simulink model "Traffic_Light_ROS2_demo"  (R2024b)
settings: Solver=FixedStepAuto  StartTime=0.0  StopTime=60  FixedStep=0.1  MaxStep=0.05  RelTol=1e-3
model workspace (MAT data in the model file):
  SL_ROS_VariableLengthArrays_MaxSizes : object (value not decoded)
undefined symbols (not defined in the file or in its folder): brake, gear, hand_brake, manual_gear_shift, reverse, steer, throttle
libraries: ros2lib x9, visionsinks x1
(part 2 of 2)

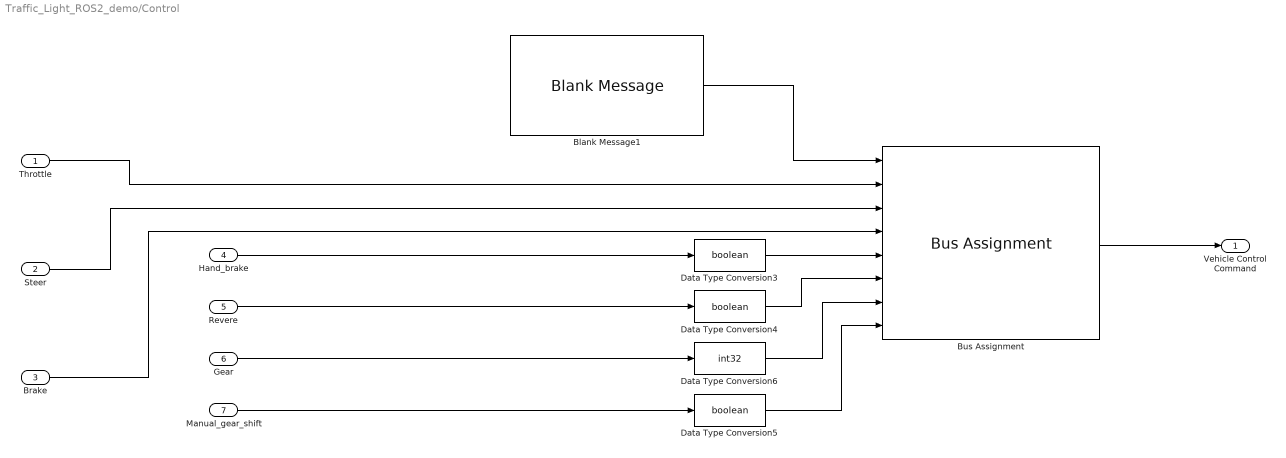
== system Traffic_Light_ROS2_demo/Control ==
  Throttle : Inport
  Steer : Inport  Port=2
  Brake : Inport  Port=3
  Hand_brake : Inport  Port=4
  Revere : Inport  Port=5
  Gear : Inport  Port=6
  Manual_gear_shift : Inport  Port=7
  Blank Message1 : ros2lib/Blank Message  messageClass=Message  entityType=carla_msgs/CarlaEgoVehicleControl  messageType=carla_msgs/CarlaEgoVehicleControl  SampleTime=inf
  Bus Assignment : BusAssignment  AssignedSignals=throttle,steer,brake,hand_brake,reverse,gear,manual_gear_shift
  Data Type Conversion3 : DataTypeConversion  OutDataTypeStr=boolean  SaturateOnIntegerOverflow=off  RndMeth=Floor
  Data Type Conversion4 : DataTypeConversion  OutDataTypeStr=boolean  SaturateOnIntegerOverflow=off  RndMeth=Floor
  Data Type Conversion5 : DataTypeConversion  OutDataTypeStr=boolean  SaturateOnIntegerOverflow=off  RndMeth=Floor
  Data Type Conversion6 : DataTypeConversion  OutDataTypeStr=int32  SaturateOnIntegerOverflow=off  RndMeth=Floor
  Vehicle Control Command : Outport
  wires:
  Data Type Conversion5/1 -> Bus Assignment/8
  Data Type Conversion6/1 -> Bus Assignment/7
  Blank Message1/1 -> Bus Assignment/1
  Data Type Conversion4/1 -> Bus Assignment/6
  Data Type Conversion3/1 -> Bus Assignment/5
  Throttle/1 -> Bus Assignment/2
  Manual_gear_shift/1 -> Data Type Conversion5/1
  Bus Assignment/1 -> Vehicle Control Command/1
  Revere/1 -> Data Type Conversion4/1
  Steer/1 -> Bus Assignment/3
  Brake/1 -> Bus Assignment/4
  Hand_brake/1 -> Data Type Conversion3/1
  Gear/1 -> Data Type Conversion6/1

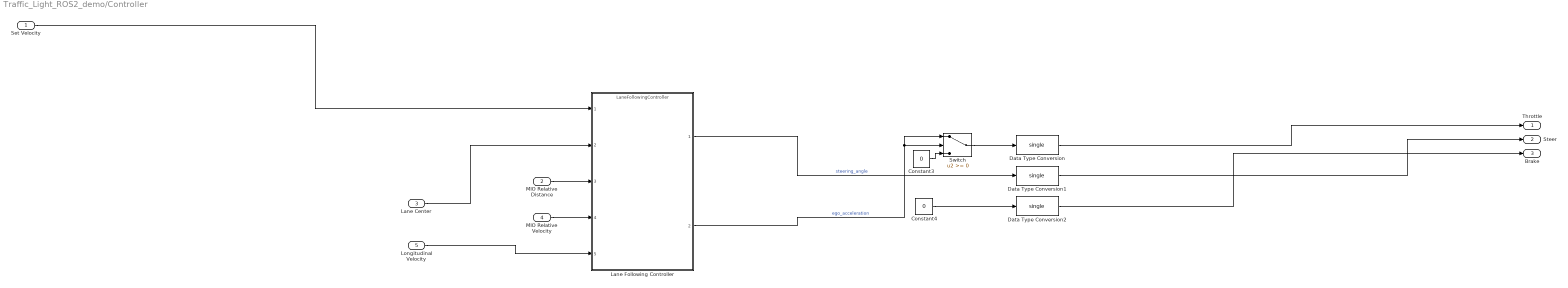
== system Traffic_Light_ROS2_demo/Controller ==
  Set Velocity : Inport
  MIO Relative Distance : Inport  Port=2
  Lane Center : Inport  Port=3
  MIO Relative Velocity : Inport  Port=4
  Longitudinal Velocity : Inport  Port=5
  Constant3 : Constant  Value=0
  Constant4 : Constant  Value=0
  Data Type Conversion : DataTypeConversion  OutDataTypeStr=single  SaturateOnIntegerOverflow=off  RndMeth=Floor
  Data Type Conversion1 : DataTypeConversion  OutDataTypeStr=single  SaturateOnIntegerOverflow=off  RndMeth=Floor
  Data Type Conversion2 : DataTypeConversion  OutDataTypeStr=single  SaturateOnIntegerOverflow=off  RndMeth=Floor
  Lane Following Controller : ModelReference  ModelNameDialog=LaneFollowingController  SimulationMode=Normal  CodeInterface=Top model  ModelReferenceVersion=10.13
  Switch : Switch  SaturateOnIntegerOverflow=off  InputSameDT=off
  Throttle : Outport
  Steer : Outport  Port=2
  Brake : Outport  Port=3
  wires:
  Set Velocity/1 -> Lane Following Controller/1
  Longitudinal Velocity/1 -> Lane Following Controller/5
  Constant3/1 -> Switch/3
  Lane Following Controller/1 -> Data Type Conversion1/1  "steering_angle"
  Data Type Conversion2/1 -> Brake/1
  MIO Relative Velocity/1 -> Lane Following Controller/4
  Data Type Conversion1/1 -> Steer/1
  Lane Center/1 -> Lane Following Controller/2
  Switch/1 -> Data Type Conversion/1
  Constant4/1 -> Data Type Conversion2/1
  MIO Relative Distance/1 -> Lane Following Controller/3
  Lane Following Controller/2 -> Switch/1, Switch/2  "ego_acceleration"
  Data Type Conversion/1 -> Throttle/1

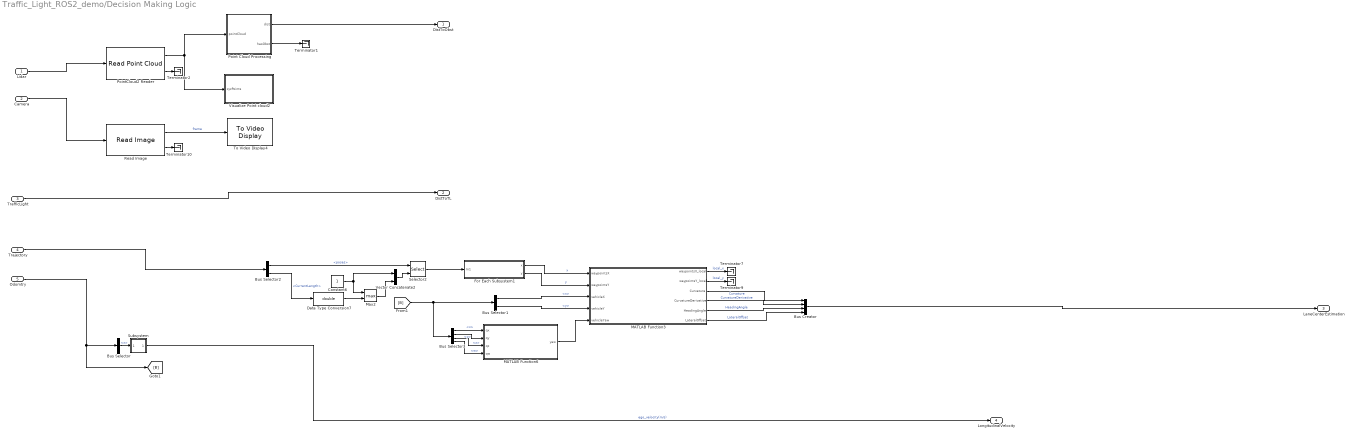
== system Traffic_Light_ROS2_demo/Decision Making Logic ==
  Lidar : Inport
  Camera : Inport  Port=2
  TrafficLight : Inport  Port=3
  Trajectory : Inport  Port=4
  Odomtry : Inport  Port=5
  Bus Creator : BusCreator  Inputs=4
  Bus Selector : BusSelector  OutputSignals=twist.twist.linear.x
  Bus Selector1 : BusSelector  OutputSignals=pose.pose.position.x,pose.pose.position.y
  Bus Selector2 : BusSelector  OutputSignals=poses,poses_SL_Info.CurrentLength
  Bus Selector3 : BusSelector  OutputSignals=pose.pose.orientation.x,pose.pose.orientation.y,pose.pose.orientation.z,pose.pose.orientation.w
  Constant6 : Constant  SampleTime=-1
  Data Type Conversion7 : DataTypeConversion  OutDataTypeStr=double  SaturateOnIntegerOverflow=off  RndMeth=Floor
  For Each Subsystem1 : Subsystem  TreatAsAtomicUnit=on
  MATLAB Function3 : MATLAB Function  TreatAsAtomicUnit=on
  MATLAB Function6 : MATLAB Function  TreatAsAtomicUnit=on
  Max2 : MinMax  Function=max  Inputs=2
  Point Cloud Processing : Subsystem
  PointCloud2 Reader : ros2lib/Read Point Cloud  MaximumPointCloudSize=[1, 8292]  PreserveStructure=off  ShowRGBOutput=off  ShowIntensityOutput=off  ShowErrorCodeOutput=on  VariableSizeOutputs=off
  Read Image : ros2lib/Read Image  MaximumImageSize=[600, 800]  ImageEncoding=bgra8  ShowAlphaOutput=off  ShowErrorCodeOutput=on  VariableSizeOutputs=off
  Selector2 : Selector  IndexOptions=Starting and ending indices (port)  Indices=1  OutputSizes=1  RuntimeRangeChecks=on
  Subsystem : Subsystem
  Terminator{1..2,7,9..10} (5 alike) : Terminator
  To Video Display4 : visionsinks/To Video Display  windowSizeMode=Normal  openAtMdlStart=on  fullScreen=off  videoWindowX=536805376  videoWindowY=536805376  saveWindowSize=off  videoWindowWidth=1395  videoWindowHeight=752  inputColorFormat=RGB  inputType=Obsolete  imagePorts=One multidimensional signal  OutputDevice=On-screen video monitor  dataOrg=Column-major  isWindowOpen=off
  Vector Concatenate2 : Concatenate
  Visualize Point cloud2 : MATLAB Function  StopFcn=|  TreatAsAtomicUnit=on
      | playerFigure = findall(groot,'type','figure','name','Point Cloud Player');
      | 
      | if ~isempty(playerFigure)
      |     playerFigure = playerFigure(end);
      |     if isvalid(playerFigure)
      |         close(playerFigure);
      |     end
      | end
  DistToObst : Outport
  DistToTL : Outport  Port=2
  LaneCenterEstimation : Outport  Port=3
  LongitudinalVelocity : Outport  Port=4
  wires:
  MATLAB Function3/5(HeadingAngle) -> Bus Creator/3  "HeadingAngle"
  Read Image/2 -> Terminator10/1
  Subsystem/1(Out1) -> LongitudinalVelocity/1  "ego_velocity(m/s)"
  PointCloud2 Reader/2 -> Terminator2/1
  MATLAB Function3/3(Curvature) -> Bus Creator/1  "Curvature"
  Bus Selector3/1 -> MATLAB Function6/1(qx)  "<x>"
  PointCloud2 Reader/1 -> Visualize Point cloud2/1(xyzPoints), Point Cloud Processing/1(pointCloud)
  Odomtry/1 -> [B], Bus Selector/1
  Constant6/1 -> Vector Concatenate2/1, Max2/1
  Read Image/1 -> To Video Display4/1  "frame"
  Data Type Conversion7/1 -> Max2/2
  For Each Subsystem1/1(x) -> MATLAB Function3/1(waypointsX)  "x"
  Bus Selector2/1 -> Selector2/1  "<poses>"
  Bus Selector3/3 -> MATLAB Function6/3(qz)  "<z>"
  Bus Selector2/2 -> Data Type Conversion7/1  "<CurrentLength>"
  Point Cloud Processing/2(hasObst) -> Terminator1/1
  MATLAB Function3/6(LateralOffset) -> Bus Creator/4  "LateralOffset"
  Trajectory/1 -> Bus Selector2/1
  Bus Selector3/4 -> MATLAB Function6/4(qw)  "<w>"
  Selector2/1 -> For Each Subsystem1/1(In1)
  MATLAB Function3/2(waypointsY_local) -> Terminator9/1  "local_y"
  Lidar/1 -> PointCloud2 Reader/1
  MATLAB Function6/1(yaw) -> MATLAB Function3/5(vehicleYaw)
  Point Cloud Processing/1(dist) -> DistToObst/1
  Camera/1 -> Read Image/1
  Bus Selector3/2 -> MATLAB Function6/2(qy)  "<y>"
  Vector Concatenate2/1 -> Selector2/2
  [B] -> Bus Selector1/1, Bus Selector3/1
  Bus Selector1/2 -> MATLAB Function3/4(vehicleY)  "<y>"
  Bus Creator/1 -> LaneCenterEstimation/1
  MATLAB Function3/1(waypointsX_local) -> Terminator7/1  "local_x"
  Bus Selector/1 -> Subsystem/1(In1)  "<x>"
  Max2/1 -> Vector Concatenate2/2
  MATLAB Function3/4(CurvatureDerivative) -> Bus Creator/2  "CurvatureDerivative"
  For Each Subsystem1/2(y) -> MATLAB Function3/2(waypointsY)  "y"
  Bus Selector1/1 -> MATLAB Function3/3(vehicleX)  "<x>"
  TrafficLight/1 -> DistToTL/1

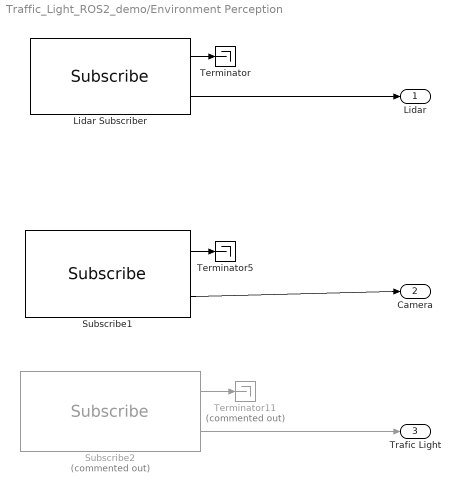
== system Traffic_Light_ROS2_demo/Environment Perception ==
  Lidar Subscriber : ros2lib/Subscribe  topicSource=Select from ROS network  topic=/carla/hero/lidar  messageType=sensor_msgs/PointCloud2  sampleTime=-1  QOSHistory=Keep last  QOSDepth=1  QOSReliability=Reliable  QOSDurability=Volatile  QOSDeadline=Inf  QOSLifespan=Inf  QOSLiveliness=Automatic  QOSLeaseDuration=Inf  QOSAvoidROSNamespaceConventions=off
  Subscribe1 : ros2lib/Subscribe  topicSource=Select from ROS network  topic=/carla/hero/rgb_front/image  messageType=sensor_msgs/Image  sampleTime=-1  QOSHistory=Keep last  QOSDepth=1  QOSReliability=Reliable  QOSDurability=Volatile  QOSDeadline=Inf  QOSLifespan=Inf  QOSLiveliness=Automatic  QOSLeaseDuration=Inf  QOSAvoidROSNamespaceConventions=off
  Subscribe2 : ros2lib/Subscribe  Commented=on  topicSource=Select from ROS network  topic=/carla/hero/traffic_light_in_front  messageType=carla_msgs/TrafficLightInfo  sampleTime=-1  QOSHistory=Keep last  QOSDepth=1  QOSReliability=Reliable  QOSDurability=Transient local  QOSDeadline=Inf  QOSLifespan=Inf  QOSLiveliness=Automatic  QOSLeaseDuration=Inf  QOSAvoidROSNamespaceConventions=off
  Terminator : Terminator
  Terminator11 : Terminator  Commented=on
  Terminator5 : Terminator
  Lidar : Outport
  Camera : Outport  Port=2
  Trafic Light : Outport  Port=3
  wires:
  Subscribe2/1 -> Terminator11/1
  Lidar Subscriber/1 -> Terminator/1
  Subscribe1/1 -> Terminator5/1
  Subscribe2/2 -> Trafic Light/1
  Lidar Subscriber/2 -> Lidar/1
  Subscribe1/2 -> Camera/1

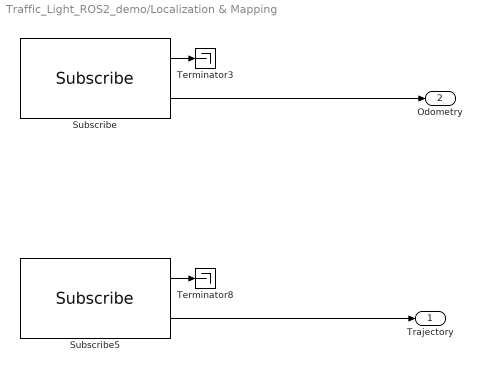
== system Traffic_Light_ROS2_demo/Localization & Mapping ==
  Subscribe : ros2lib/Subscribe  topicSource=Select from ROS network  topic=/carla/hero/odometry  messageType=nav_msgs/Odometry  sampleTime=-1  QOSHistory=Keep last  QOSDepth=1  QOSReliability=Reliable  QOSDurability=Volatile  QOSDeadline=Inf  QOSLifespan=Inf  QOSLiveliness=Automatic  QOSLeaseDuration=Inf  QOSAvoidROSNamespaceConventions=off
  Subscribe5 : ros2lib/Subscribe  topicSource=Select from ROS network  topic=/carla/hero/waypoints  messageType=nav_msgs/Path  sampleTime=-1  QOSHistory=Keep last  QOSDepth=1  QOSReliability=Reliable  QOSDurability=Transient local  QOSDeadline=Inf  QOSLifespan=Inf  QOSLiveliness=Automatic  QOSLeaseDuration=Inf  QOSAvoidROSNamespaceConventions=off
  Terminator3 : Terminator
  Terminator8 : Terminator
  Trajectory : Outport
  Odometry : Outport  Port=2
  wires:
  Subscribe5/1 -> Terminator8/1
  Subscribe/1 -> Terminator3/1
  Subscribe5/2 -> Trajectory/1
  Subscribe/2 -> Odometry/1

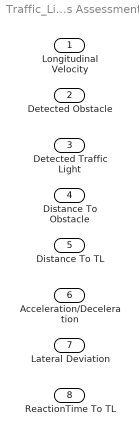
== system Traffic_Light_ROS2_demo/Metrics Assessment ==
  Longitudinal Velocity : Inport
  Detected Obstacle : Inport  Port=2
  Detected Traffic Light : Inport  Port=3
  Distance To Obstacle : Inport  Port=4
  Distance To TL : Inport  Port=5
  Acceleration/Deceleration : Inport  Port=6
  Lateral Deviation : Inport  Port=7
  ReactionTime To TL : Inport  Port=8

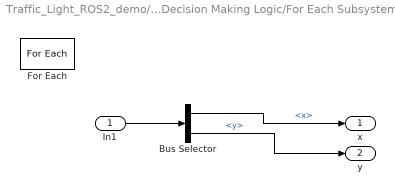
== system Traffic_Light_ROS2_demo/Decision Making Logic/For Each Subsystem1 ==
  In1 : Inport  Partition=on  PartitionDimension=1  PartitionWidth=1  PartitionOffset=0
  Bus Selector : BusSelector  OutputSignals=pose.position.x,pose.position.y
  For Each : ForEach  DisableCoverage=on
  x : Outport  ConcatenationDimension=1
  y : Outport  Port=2  ConcatenationDimension=1
  wires:
  In1/1 -> Bus Selector/1
  Bus Selector/1 -> x/1  "<x>"
  Bus Selector/2 -> y/1  "<y>"

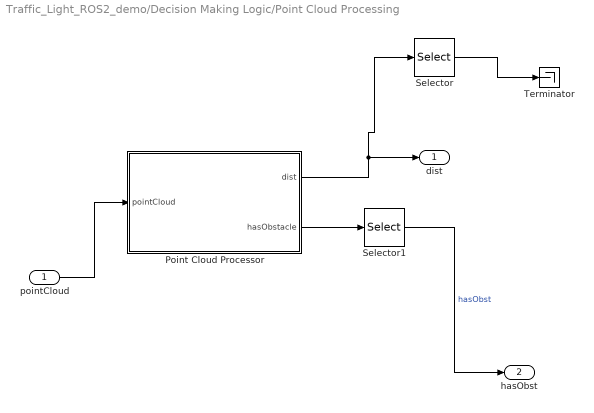
== system Traffic_Light_ROS2_demo/Decision Making Logic/Point Cloud Processing ==
  pointCloud : Inport
  Point Cloud Processor : MATLAB Function  TreatAsAtomicUnit=on
  Selector : Selector  InputPortWidth=10000  IndexOptions=Index vector (dialog)  Indices=1  OutputSizes=1
  Selector1 : Selector  IndexOptions=Index vector (dialog)  Indices=1  OutputSizes=1
  Terminator : Terminator
  dist : Outport
  hasObst : Outport  Port=2
  wires:
  Point Cloud Processor/2(hasObstacle) -> Selector1/1
  Selector/1 -> Terminator/1
  pointCloud/1 -> Point Cloud Processor/1(pointCloud)
  Point Cloud Processor/1(dist) -> dist/1, Selector/1
  Selector1/1 -> hasObst/1  "hasObst"

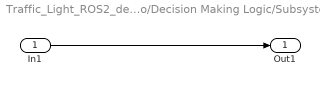
== system Traffic_Light_ROS2_demo/Decision Making Logic/Subsystem ==
  In1 : Inport
  Out1 : Outport
  wires:
  In1/1 -> Out1/1

== matlab function Traffic_Light_ROS2_demo/Decision Making Logic/Point Cloud Processing/Point Cloud Processor ==
  data: pointCloud input; dist output size=[10000,1]; hasObstacle output double
function [dist, hasObstacle] = detectObstacles(pointCloud)
% Detect obstacles from a point cloud and calculate the closest distance.

% Inputs:
%   pointCloud - Nx3 array of [x, y, z] points (point cloud data)
%   lateralRange - Lateral range of interest (meters)
%   zGroundThreshold - Minimum z-value to exclude ground points (meters)

% Outputs:
%   dist - Closest distance to an obstacle (scalar, meters)
%   hasObstacle - Boolean flag indicating if an obstacle is detected

% Initialize outputs
dist = single(inf); % Default to infinity
hasObstacle = 0;


% Check if pointCloud is empty
if isempty(pointCloud)
    return; % Return default outputs
end

% Extract coordinates
x = pointCloud(:, 1); % Forward (X) axis
y = pointCloud(:, 2); % Lateral (Y) axis
z = pointCloud(:, 3); % Vertical (Z) axis

lateralRange = 3;
zGroundThreshold = -2;

% Filter points within region of interest (ROI)
% ROI Criteria:
% - In front of the ego vehicle: x > 0
% - Within lateral range: |y| < lateralRange
% - Above ground: z > zGroundThreshold
isInROI = (x > 0) & (abs(y) < lateralRange) & (z > zGroundThreshold);

% Apply filter
filteredPoints = pointCloud(isInROI, :);

% Compute the closest distance
if ~isempty(filteredPoints)
    % Compute Euclidean distances in the X-Y plane
    % distances = sqrt(filteredPoints(:, 1).^2 + filteredPoints(:, 2).^2); 
    % dist = min(distances); % Find the closest distance
    dist = mean(filteredPoints(:, 1));
    hasObstacle = 1; % Set obstacle flag to true
end

end

== matlab function Traffic_Light_ROS2_demo/Decision Making Logic/Visualize Point cloud2 ==
  data: xyzPoints input
function VisualizePointCloud(xyzPoints)
%VisualizePointCloud Display point cloud

coder.extrinsic('isOpen', 'pcplayer')

persistent player;

if isempty(player)
    % Configure axes limits
    xlimits = [-90 90];
    ylimits = [-90 90];
    zlimits = [ -5 40];
    
    % Create a streaming Lidar viewer
    player = pcplayer(xlimits, ylimits, zlimits);
end

if ~isempty(player) && isOpen(player)
    view(player, xyzPoints);
end

== matlab function Traffic_Light_ROS2_demo/Decision Making Logic/MATLAB Function3 ==
  data: waypointsX input; waypointsX_local output; waypointsY input; vehicleX input; vehicleY input; vehicleYaw input; waypointsY_local output; Curvature output; CurvatureDerivative output; HeadingAngle output; LateralOffset output
function [waypointsX_local, waypointsY_local, Curvature, CurvatureDerivative, HeadingAngle, LateralOffset] = computeLaneCenter(waypointsX, waypointsY, vehicleX, vehicleY, vehicleYaw)
    % Inputs:
    %   waypointsX: X coordinates of the waypoints (Nx1 vector)
    %   waypointsY: Y coordinates of the waypoints (Nx1 vector)
    %   vehicleX: X coordinate of the vehicle
    %   vehicleY: Y coordinate of the vehicle
    %   vehicleYaw: Vehicle orientation (yaw) in radians
    % Outputs:
    %   Curvature: Lane curvature at the vehicle's position
    %   CurvatureDerivative: Rate of change of curvature
    %   HeadingAngle: Lane heading angle at the vehicle's position
    %   LateralOffset: Distance from the vehicle to the lane center (meters)

    % Ensure inputs are column vectors
    waypointsX = waypointsX(:);
    waypointsY = waypointsY(:);

    % Transform waypoints to local vehicle coordinates
    dx = waypointsX - vehicleX;
    dy = waypointsY - vehicleY;
    waypointsX_local = dx * cos(vehicleYaw) + dy * sin(vehicleYaw);
    waypointsY_local = -dx * sin(vehicleYaw) + dy * cos(vehicleYaw);

    % Filter waypoints to include only those ahead of the vehicle
    maxRange = 25; % Limit to 50 meters ahead
    rangeIdx = waypointsX_local > 0 & waypointsX_local < maxRange;
    waypointsX_local = waypointsX_local(rangeIdx);
    waypointsY_local = waypointsY_local(rangeIdx);

    % Ensure enough points are available for fitting
    if numel(waypointsX_local) < 3
        % Not enough points to compute reliably
        Curvature = single(0);
        CurvatureDerivative = single(0);
        HeadingAngle = single(0);
        LateralOffset = single(0);
        return;
    end

    % Fit a 2nd-order polynomial to the filtered waypoints
    polyCoeffs = polyfit(waypointsX_local, waypointsY_local, 2); % y = ax^2 + bx + c
    a = polyCoeffs(1); % Quadratic coefficient
    b = polyCoeffs(2); % Linear coefficient
    c = polyCoeffs(3); % Constant term

    % Curvature: k = 2a / (1 + b^2)^(3/2)
    Curvature = single(2 * a / (1 + b^2)^(3/2));

    % Curvature Derivative: k' = -6a^2b / (1 + b^2)^(5/2)
    CurvatureDerivative = single(-6 * a^2 * b / (1 + b^2)^(5/2));

    % Heading Angle: theta = atan(b)
    HeadingAngle = single(atan(b));

    % Lateral Offset: y = ax^2 + bx + c at x = 0
    LateralOffset = single(c); % Since x_vehicle_local = 0
    % 
    % % Debugging Outputs (optional)
    % disp('Polynomial Coefficients (a, b, c):');
    % disp(polyCoeffs);
    % disp('Curvature:');
    % disp(Curvature);
    % disp('Curvature Derivative:');
    % disp(CurvatureDerivative);
    % disp('Heading Angle:');
    % disp(HeadingAngle);
    % disp('Lateral Offset:');
    % disp(LateralOffset);
end

== matlab function Traffic_Light_ROS2_demo/Decision Making Logic/MATLAB Function6 ==
  data: qx input; yaw output; qy input; qz input; qw input
function yaw = quaternionToYaw(qx, qy, qz, qw)
    % Convert quaternion (qx, qy, qz, qw) to yaw angle in radians
    % This formula is based on the standard conversion from quaternion to Euler angles

    % Calculate yaw from quaternion
    siny_cosp = 2 * (qw * qz + qx * qy);
    cosy_cosp = 1 - 2 * (qy^2 + qz^2);
    yaw = atan2(siny_cosp, cosy_cosp); % result is in radians
end
